simulink model "AWFG_2022b"  (R2021b)
settings: Solver=FixedStepDiscrete  StartTime=0.0  StopTime=2e-3  FixedStep=2e-8  RelTol=1e-3
settings Model: Creator=steal  LastModifiedBy=estra
settings SolverCC: AlgebraicLoopSolver=TrustRegion
settings DataIOCC: ReturnWorkspaceOutputs=off
settings OptimizationCC: DefaultParameterBehavior=Inlined  PassReuseOutputArgsAs=Individual arguments  EfficientTunableParamExpr=on
settings DebuggingCC: ParameterTunabilityLossMsg=error  BusObjectLabelMismatch=error  SFMachineParentedDataDiag=warning  ArithmeticOperatorsInVariantConditions=warning
settings SFSimCC: SimUseLocalCustomCode=off  MATLABDynamicMemAlloc=off  CustomCodeUndefinedFunction=UseInterfaceOnly
settings RTWCC: Description=Embedded Coder  SystemTargetFile=ert.tlc  GenCodeOnly=on  TemplateMakefile=ert_default_tmf  GenerateReport=on  RTWUseLocalCustomCode=off  IncludeHyperlinkInReport=on  LaunchReport=on  GenerateTraceInfo=on  GenerateTraceReport=on  GenerateTraceReportSl=on  GenerateTraceReportSf=on  GenerateTraceReportEml=on
settings CodeAppCC: ForceParamTrailComments=on  IgnoreCustomStorageClasses=off  OperatorAnnotations=on  SimulinkDataObjDesc=on  SFDataObjDesc=on  InsertBlockDesc=on
settings ERTTargetCC: TargetLangStandard=C99 (ISO)  GenerateSampleERTMain=on  SupportVariableSizeSignals=on  InlinedParameterPlacement=NonHierarchical  ERTCustomFileTemplate=example_file_process.tlc

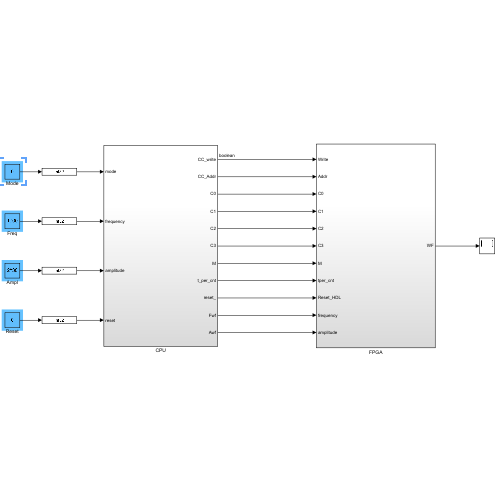
[thumbnail: Simulink's stored preview of the top-level diagram]
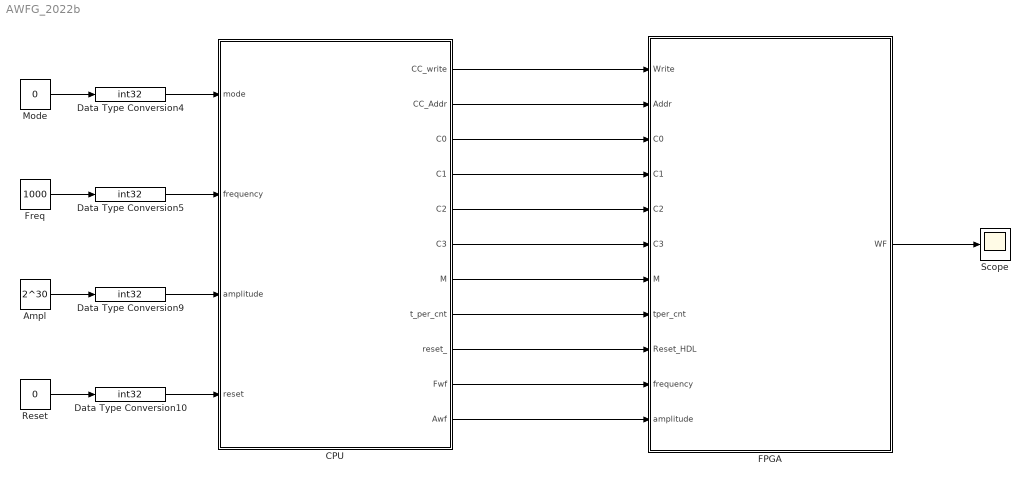
== system AWFG_2022b ==
  Ampl : Constant  Value=2^30  OutDataTypeStr=single  SampleTime=-1
  CPU : Subsystem
  Data Type Conversion{4..5,9..10} (4 alike) : DataTypeConversion  OutDataTypeStr=int32
  FPGA : Subsystem
  Freq : Constant  Value=1000  OutDataTypeStr=single  SampleTime=-1
  Mode : Constant  Value=0  OutDataTypeStr=single  SampleTime=-1
  Reset : Constant  Value=0  OutDataTypeStr=single  SampleTime=-1
  Scope : Scope
  wires:
  CPU/3(C0) -> FPGA/3(C0)
  CPU/2(CC_Addr) -> FPGA/2(Addr)
  CPU/1(CC_write) -> FPGA/1(Write)
  CPU/4(C1) -> FPGA/4(C1)
  CPU/5(C2) -> FPGA/5(C2)
  CPU/6(C3) -> FPGA/6(C3)
  Ampl/1 -> Data Type Conversion9/1
  Mode/1 -> Data Type Conversion4/1
  Freq/1 -> Data Type Conversion5/1
  Reset/1 -> Data Type Conversion10/1
  Data Type Conversion4/1 -> CPU/1(mode)
  Data Type Conversion10/1 -> CPU/4(reset)
  Data Type Conversion5/1 -> CPU/2(frequency)
  CPU/7(M) -> FPGA/7(M)
  CPU/8(t_per_cnt) -> FPGA/8(tper_cnt)
  FPGA/1(WF) -> Scope/1
  Data Type Conversion9/1 -> CPU/3(amplitude)
  CPU/11(Awf) -> FPGA/11(amplitude)
  CPU/9(reset_) -> FPGA/9(Reset_HDL)
  CPU/10(Fwf) -> FPGA/10(frequency)

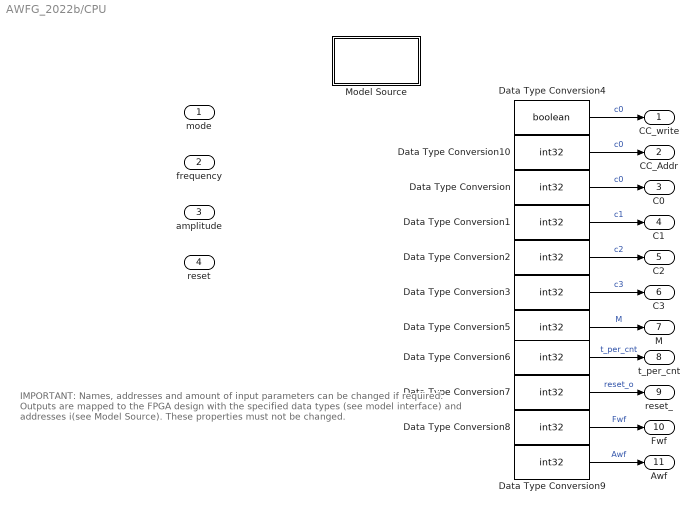
== system AWFG_2022b/CPU ==
  note: IMPORTANT:
      | Names, addresses and amount of input parameters can be changed if required.
      |
      | Outputs are mapped to the FPGA design with the specified data types (see model interface) and addresses i(see Model Source). These properties must not be changed.
  mode : Inport
  frequency : Inport  Port=2
  amplitude : Inport  Port=3
  reset : Inport  Port=4
  Data Type Conversion{,1..3,5..10} (10 alike) : DataTypeConversion  OutDataTypeStr=int32
  Data Type Conversion4 : DataTypeConversion  OutDataTypeStr=boolean
  Model Source : Subsystem  mask(Model Source){ShowInLibBrowser=0}
      mask prompts: ShowInLibBrowser "Simulink:masks:CustCodeMaskParam1_MP"
      settings: CopyFcn=cccopyfcn(gcb)  OpenFcn=ccopenfcn('Model Source')
      mask Help: eval('feval(''rtwprivate'',''rtwhelpview'',''rtw_model_source_block'')');
      mask Display: disp('Model\nSource');
  CC_write : Outport  OutDataTypeStr=boolean  VectorParamsAs1DForOutWhenUnconnected=off
  CC_Addr : Outport  Port=2  VectorParamsAs1DForOutWhenUnconnected=off
  C0 : Outport  Port=3  VectorParamsAs1DForOutWhenUnconnected=off
  C1 : Outport  Port=4  VectorParamsAs1DForOutWhenUnconnected=off
  C2 : Outport  Port=5  VectorParamsAs1DForOutWhenUnconnected=off
  C3 : Outport  Port=6  VectorParamsAs1DForOutWhenUnconnected=off
  M : Outport  Port=7  VectorParamsAs1DForOutWhenUnconnected=off
  t_per_cnt : Outport  Port=8  VectorParamsAs1DForOutWhenUnconnected=off
  reset_ : Outport  Port=9  VectorParamsAs1DForOutWhenUnconnected=off
  Fwf : Outport  Port=10  VectorParamsAs1DForOutWhenUnconnected=off
  Awf : Outport  Port=11  VectorParamsAs1DForOutWhenUnconnected=off
  wires:
  Data Type Conversion/1 -> C0/1  "c0"
  Data Type Conversion1/1 -> C1/1  "c1"
  Data Type Conversion2/1 -> C2/1  "c2"
  Data Type Conversion3/1 -> C3/1  "c3"
  Data Type Conversion4/1 -> CC_write/1  "c0"
  Data Type Conversion5/1 -> M/1  "M"
  Data Type Conversion6/1 -> t_per_cnt/1  "t_per_cnt"
  Data Type Conversion7/1 -> reset_/1  "reset_o"
  Data Type Conversion8/1 -> Fwf/1  "Fwf"
  Data Type Conversion9/1 -> Awf/1  "Awf"
  Data Type Conversion10/1 -> CC_Addr/1  "c0"

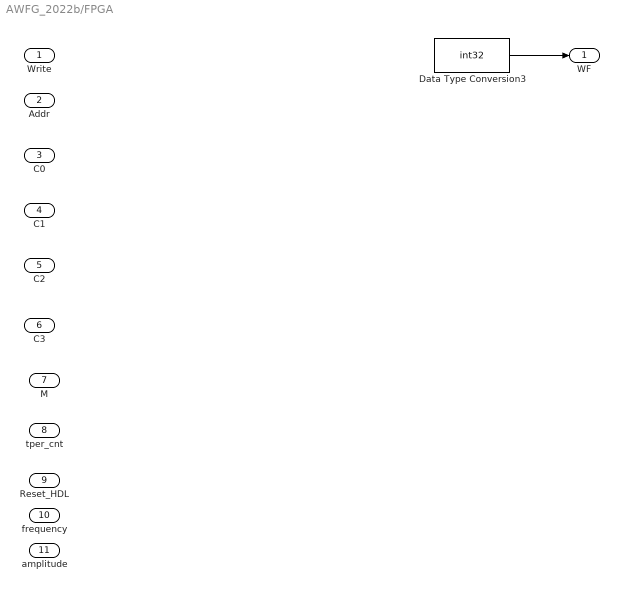
== system AWFG_2022b/FPGA ==
  Write : Inport
  Addr : Inport  Port=2
  C0 : Inport  Port=3
  C1 : Inport  Port=4
  C2 : Inport  Port=5
  C3 : Inport  Port=6
  M : Inport  Port=7
  tper_cnt : Inport  Port=8
  Reset_HDL : Inport  Port=9
  frequency : Inport  Port=10
  amplitude : Inport  Port=11
  Data Type Conversion3 : DataTypeConversion  OutDataTypeStr=int32
  WF : Outport  VectorParamsAs1DForOutWhenUnconnected=off
  wires:
  Data Type Conversion3/1 -> WF/1

== system AWFG_2022b/CPU/Model Source ==
